simulink model "Flight_Physics_forTrim"  (R2017b)
settings: Solver=ode4  StartTime=0  StopTime=50  FixedStep=Ts  RelTol=1e-3
undefined symbols (not defined in the file or in its folder): Configuration, FOR_LDG_R_B, g, MOM_LDG_R_B, Sim_Control, Ts
libraries: MathLibrary x3, shared6dof x1
settings Model: Creator=zht  LastModifiedBy=zht
settings DataIOCC: SaveFormat=StructureWithTime
settings OptimizationCC: BlockReduction=off  OptimizeBlockIOStorage=off  BufferReuse=off  GlobalBufferReuse=off  ExpressionFolding=off  LocalBlockOutputs=off
settings DebuggingCC: AlgebraicLoopMsg=none  UnconnectedInputMsg=none  UnconnectedOutputMsg=none  UnconnectedLineMsg=none

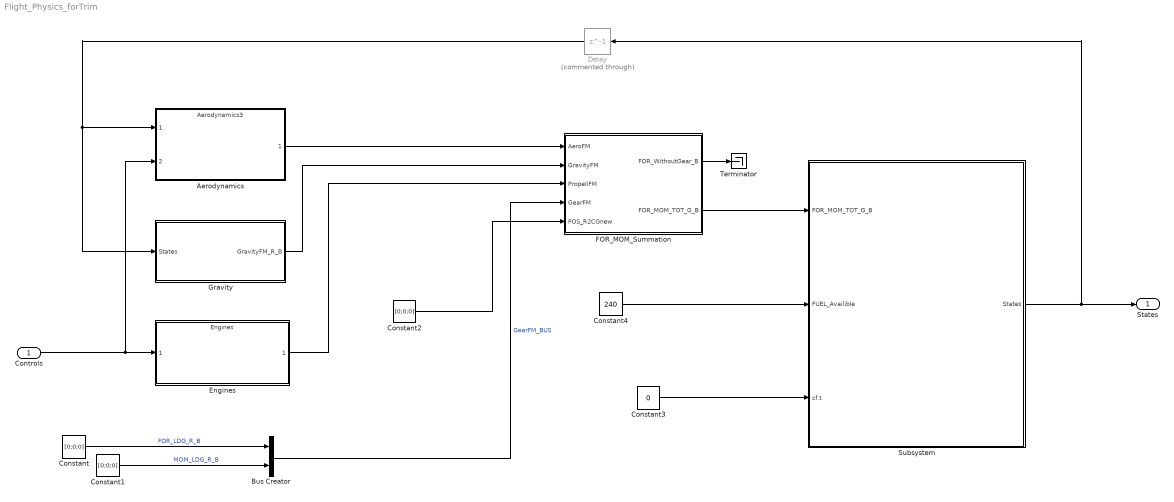
== system Flight_Physics_forTrim ==
  Controls : Inport  OutDataTypeStr=Bus: Controls_CMD_BUS
  Aerodynamics : ModelReference  ModelNameDialog=Aerodynamics3.slx  SimulationMode=Normal  ModelReferenceVersion=1.35
  Bus Creator : BusCreator  Inputs=FOR_LDG_R_B,MOM_LDG_R_B  OutDataTypeStr=Bus: GearFM_BUS  NonVirtualBus=on
  Constant : Constant  Value=[0;0;0]
  Constant1 : Constant  Value=[0;0;0]
  Constant2 : Constant  Value=[0;0;0]
  Constant3 : Constant  Value=0
  Constant4 : Constant  Value=240
  Delay : Delay  Commented=through  DelayLength=1
  Engines : ModelReference  ModelNameDialog=Engines.slx  SimulationMode=Normal  ModelReferenceVersion=1.20
  FOR_MOM_Summation : Subsystem
  Gravity : Subsystem
  Subsystem : Subsystem
  Terminator : Terminator
  States : Outport  OutDataTypeStr=Bus: States_BUS
  wires:
  Controls/1 -> Aerodynamics/2, Engines/1
  Subsystem/1(States) -> States/1, Delay/1
  FOR_MOM_Summation/2(FOR_MOM_TOT_G_B) -> Subsystem/1(FOR_MOM_TOT_G_B)
  Aerodynamics/1 -> FOR_MOM_Summation/1(AeroFM)
  Gravity/1(GravityFM_R_B) -> FOR_MOM_Summation/2(GravityFM)
  Engines/1 -> FOR_MOM_Summation/3(PropellFM)
  Constant4/1 -> Subsystem/2(FUEL_Availible)
  Constant2/1 -> FOR_MOM_Summation/5(POS_R2CGnew)
  Delay/1 -> Gravity/1(States), Aerodynamics/1
  Constant1/1 -> Bus Creator/2  "MOM_LDG_R_B"
  Constant/1 -> Bus Creator/1  "FOR_LDG_R_B"
  Bus Creator/1 -> FOR_MOM_Summation/4(GearFM)  "GearFM_BUS"
  FOR_MOM_Summation/1(FOR_WithoutGear_B) -> Terminator/1
  Constant3/1 -> Subsystem/3(cf.t)

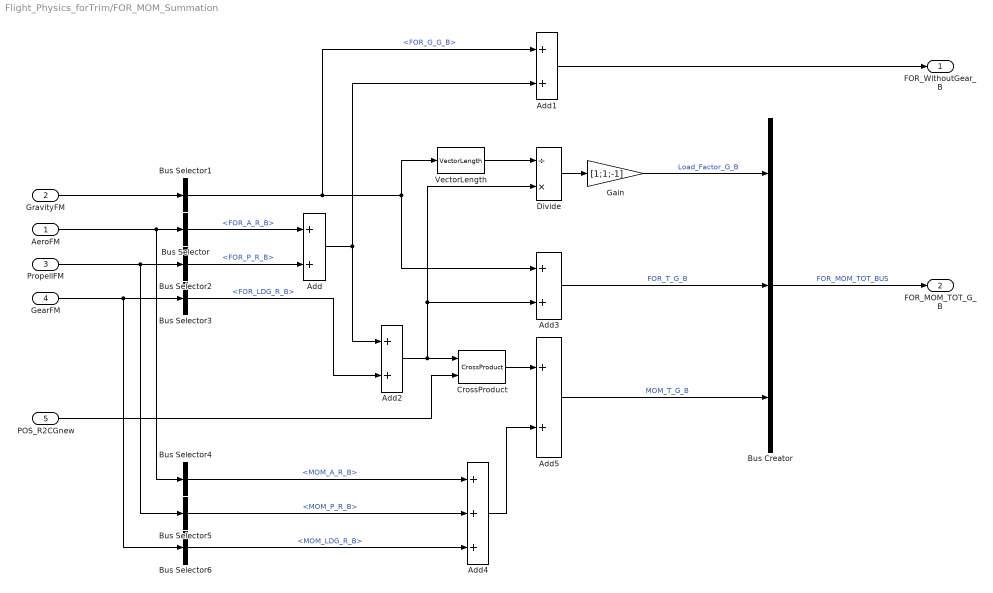
== system Flight_Physics_forTrim/FOR_MOM_Summation ==
  AeroFM : Inport  OutDataTypeStr=Bus: AeroFM_BUS
  GravityFM : Inport  Port=2  OutDataTypeStr=Bus: GravityFM_BUS
  PropellFM : Inport  Port=3  OutDataTypeStr=Bus: PropellFM_BUS
  GearFM : Inport  Port=4  OutDataTypeStr=Bus: GearFM_BUS
  POS_R2CGnew : Inport  Port=5
  Add{,1..3,5} (5 alike) : Sum
  Add4 : Sum  Inputs=+++
  Bus Creator : BusCreator  Inputs=3  OutDataTypeStr=Bus: FOR_MOM_TOT_BUS
  Bus Selector : BusSelector  OutputSignals=FOR_A_R_B
  Bus Selector1 : BusSelector  OutputSignals=FOR_G_G_B
  Bus Selector2 : BusSelector  OutputSignals=FOR_P_R_B
  Bus Selector3 : BusSelector  OutputSignals=FOR_LDG_R_B
  Bus Selector4 : BusSelector  OutputSignals=MOM_A_R_B
  Bus Selector5 : BusSelector  OutputSignals=MOM_P_R_B
  Bus Selector6 : BusSelector  OutputSignals=MOM_LDG_R_B
  CrossProduct : MathLibrary/CrossProduct
  Divide : Product  Inputs=/*
  Gain : Gain  Gain=[1;1;-1]
  VectorLength : MathLibrary/VectorLength
  FOR_WithoutGear_B : Outport
  FOR_MOM_TOT_G_B : Outport  Port=2  OutDataTypeStr=Bus: FOR_MOM_TOT_BUS
  wires:
  PropellFM/1 -> Bus Selector5/1, Bus Selector2/1
  AeroFM/1 -> Bus Selector4/1, Bus Selector/1
  GravityFM/1 -> Bus Selector1/1
  GearFM/1 -> Bus Selector3/1, Bus Selector6/1
  Bus Creator/1 -> FOR_MOM_TOT_G_B/1  "FOR_MOM_TOT_BUS"
  Add1/1 -> FOR_WithoutGear_B/1
  Bus Selector/1 -> Add/1  "<FOR_A_R_B>"
  Bus Selector2/1 -> Add/2  "<FOR_P_R_B>"
  Add/1 -> Add2/1, Add1/2
  Bus Selector1/1 -> Add1/1, VectorLength/1, Add3/1  "<FOR_G_G_B>"
  Bus Selector3/1 -> Add2/2  "<FOR_LDG_R_B>"
  Add2/1 -> CrossProduct/1, Divide/2, Add3/2
  VectorLength/1 -> Divide/1
  Divide/1 -> Gain/1
  Gain/1 -> Bus Creator/1  "Load_Factor_G_B"
  Add3/1 -> Bus Creator/2  "FOR_T_G_B"
  Bus Selector4/1 -> Add4/1  "<MOM_A_R_B>"
  Bus Selector5/1 -> Add4/2  "<MOM_P_R_B>"
  Bus Selector6/1 -> Add4/3  "<MOM_LDG_R_B>"
  CrossProduct/1 -> Add5/1
  Add4/1 -> Add5/2
  Add5/1 -> Bus Creator/3  "MOM_T_G_B"
  POS_R2CGnew/1 -> CrossProduct/2

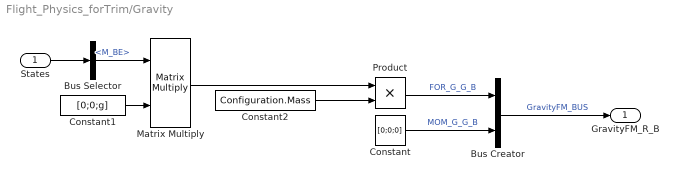
== system Flight_Physics_forTrim/Gravity ==
  States : Inport  OutDataTypeStr=Bus: States_BUS
  Bus Creator : BusCreator  Inputs=2  OutDataTypeStr=Bus: GravityFM_BUS
  Bus Selector : BusSelector  OutputSignals=M_BE
  Constant : Constant  Value=[0;0;0]
  Constant1 : Constant  Value=[0;0;g]  SampleTime=Ts
  Constant2 : Constant  Value=Configuration.Mass  SampleTime=Ts
  Matrix Multiply : Product  Multiplication=Matrix(*)
  Product : Product
  GravityFM_R_B : Outport  OutDataTypeStr=Bus: GravityFM_BUS
  wires:
  States/1 -> Bus Selector/1
  Bus Selector/1 -> Matrix Multiply/1  "<M_BE>"
  Constant1/1 -> Matrix Multiply/2
  Matrix Multiply/1 -> Product/1
  Constant2/1 -> Product/2
  Product/1 -> Bus Creator/1  "FOR_G_G_B"
  Constant/1 -> Bus Creator/2  "MOM_G_G_B"
  Bus Creator/1 -> GravityFM_R_B/1  "GravityFM_BUS"

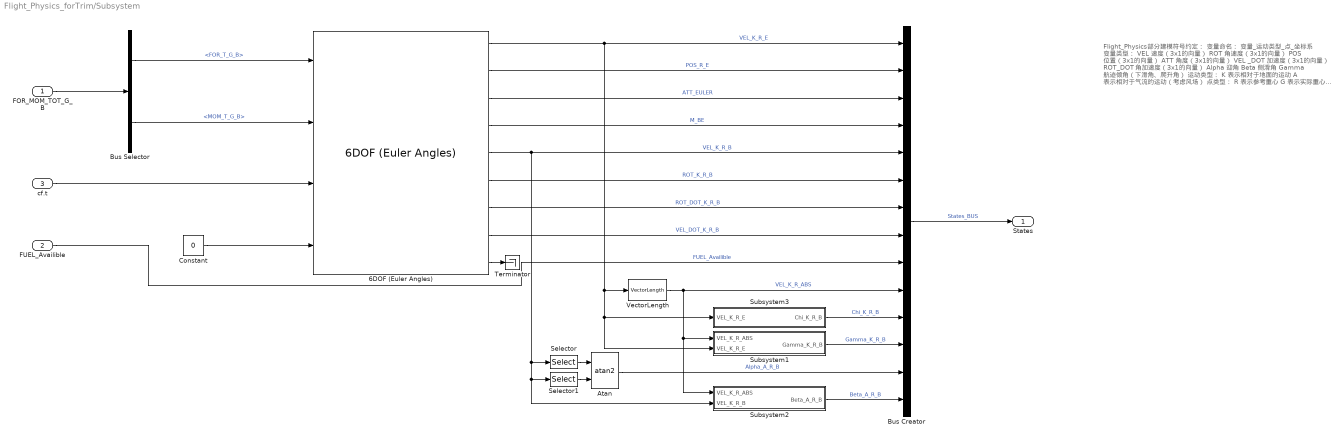
== system Flight_Physics_forTrim/Subsystem ==
  note: Flight_Physics部分建模符号约定：
      | 变量命名：
      | 变量_运动类型_点_坐标系
      |
      | 变量类型：
      | VEL 速度（3x1的向量）
      | ROT 角速度（3x1的向量）
      | POS 位置（3x1的向量）
      | ATT 角度（3x1的向量）
      | VEL _DOT 加速度（3x1的向量）
      | ROT_DOT 角加速度（3x1的向量）
      | Alpha 迎角
      | Beta 侧滑角
      | Gamma 航迹倾角（下滑角、爬升角）
      | 运动类型：
      | K 表示相对于地面的运动
      | A 表示相对于气流的运动（考虑风场）
      | 点类型：
      | R 表示参考重心
      | G 表示实际重心
      | 坐标系类型：
      | B 机体系
      | E 地面系 ABS 与坐标系无关，表示该变量的绝对值
  FOR_MOM_TOT_G_B : Inport  OutDataTypeStr=Bus: FOR_MOM_TOT_BUS
  FUEL_Availible : Inport  Port=2
  cf.t : Inport  Port=3
  6DOF (Euler Angles) : shared6dof/6DOF (Euler Angles)  units=Metric (MKS)  mtype=Simple Variable  rep=Euler Angles  xme_0=Sim_Control.init(1,:)  Vm_0=Sim_Control.init(2,:)  eul_0=Sim_Control.init(3,:)  pm_0=Sim_Control.init(4,:)  mass_0=Configuration.Mass  mass_e=Configuration.Mass_Constr  mass_f=Configuration.Mass  inertia=eye(3)  inertia_e=Configuration.Inertia_G_B  inertia_f=Configuration.Inertia_G_B  k_quat=1.0  vre_flag=on  abi_flag=off
      settings: SourceProductBaseCode=AE
  Atan : Trigonometry  Operator=atan2
  Bus Creator : BusCreator  Inputs=14  OutDataTypeStr=Bus: States_BUS
  Bus Selector : BusSelector  OutputSignals=FOR_T_G_B,MOM_T_G_B
  Constant : Constant  Value=0
  Selector : Selector  InputPortWidth=3  IndexOptions=Index vector (dialog)  Indices=[3]  OutputSizes=1
  Selector1 : Selector  InputPortWidth=3  IndexOptions=Index vector (dialog)  Indices=[1]  OutputSizes=1
  Subsystem1 : Subsystem
  Subsystem2 : Subsystem
  Subsystem3 : Subsystem
  Terminator : Terminator
  VectorLength : MathLibrary/VectorLength
  States : Outport  OutDataTypeStr=Bus: States_BUS
  wires:
  Bus Creator/1 -> States/1  "States_BUS"
  Bus Selector/2 -> 6DOF (Euler Angles)/2  "<MOM_T_G_B>"
  Bus Selector/1 -> 6DOF (Euler Angles)/1  "<FOR_T_G_B>"
  FOR_MOM_TOT_G_B/1 -> Bus Selector/1
  6DOF (Euler Angles)/1 -> VectorLength/1, Subsystem3/1(VEL_K_R_E), Subsystem1/2(VEL_K_R_E), Bus Creator/1  "VEL_K_R_E"
  6DOF (Euler Angles)/2 -> Bus Creator/2  "POS_R_E"
  6DOF (Euler Angles)/3 -> Bus Creator/3  "ATT_EULER"
  6DOF (Euler Angles)/4 -> Bus Creator/4  "M_BE"
  6DOF (Euler Angles)/5 -> Subsystem2/2(VEL_K_R_B), Selector1/1, Selector/1, Bus Creator/5  "VEL_K_R_B"
  6DOF (Euler Angles)/6 -> Bus Creator/6  "ROT_K_R_B"
  6DOF (Euler Angles)/7 -> Bus Creator/7  "ROT_DOT_K_R_B"
  6DOF (Euler Angles)/8 -> Bus Creator/8  "VEL_DOT_K_R_B"
  FUEL_Availible/1 -> Bus Creator/9  "FUEL_Availible"
  Selector/1 -> Atan/1
  Selector1/1 -> Atan/2
  Atan/1 -> Bus Creator/13  "Alpha_A_R_B"
  VectorLength/1 -> Subsystem1/1(VEL_K_R_ABS), Subsystem2/1(VEL_K_R_ABS), Bus Creator/10  "VEL_K_R_ABS"
  Subsystem1/1(Gamma_K_R_B) -> Bus Creator/12  "Gamma_K_R_B"
  Subsystem2/1(Beta_A_R_B) -> Bus Creator/14  "Beta_A_R_B"
  Subsystem3/1(Chi_K_R_B) -> Bus Creator/11  "Chi_K_R_B"
  Constant/1 -> 6DOF (Euler Angles)/4
  cf.t/1 -> 6DOF (Euler Angles)/3
  6DOF (Euler Angles)/9 -> Terminator/1

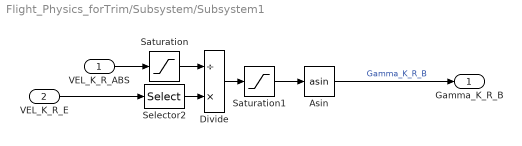
== system Flight_Physics_forTrim/Subsystem/Subsystem1 ==
  VEL_K_R_ABS : Inport
  VEL_K_R_E : Inport  Port=2
  Asin : Trigonometry  Operator=asin
  Divide : Product  Inputs=/*
  Saturation : Saturate  UpperLimit=inf  LowerLimit=0.01
  Saturation1 : Saturate  UpperLimit=1  LowerLimit=-1
  Selector2 : Selector  InputPortWidth=3  IndexOptions=Index vector (dialog)  Indices=[3]  OutputSizes=1
  Gamma_K_R_B : Outport
  wires:
  Divide/1 -> Saturation1/1
  Asin/1 -> Gamma_K_R_B/1  "Gamma_K_R_B"
  VEL_K_R_E/1 -> Selector2/1
  VEL_K_R_ABS/1 -> Saturation/1
  Selector2/1 -> Divide/2
  Saturation1/1 -> Asin/1
  Saturation/1 -> Divide/1

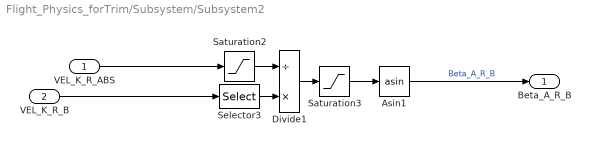
== system Flight_Physics_forTrim/Subsystem/Subsystem2 ==
  VEL_K_R_ABS : Inport
  VEL_K_R_B : Inport  Port=2
  Asin1 : Trigonometry  Operator=asin
  Divide1 : Product  Inputs=/*
  Saturation2 : Saturate  UpperLimit=inf  LowerLimit=0.01
  Saturation3 : Saturate  UpperLimit=1  LowerLimit=-1
  Selector3 : Selector  InputPortWidth=3  IndexOptions=Index vector (dialog)  Indices=[2]  OutputSizes=1
  Beta_A_R_B : Outport
  wires:
  Saturation2/1 -> Divide1/1
  Asin1/1 -> Beta_A_R_B/1  "Beta_A_R_B"
  Saturation3/1 -> Asin1/1
  Selector3/1 -> Divide1/2
  Divide1/1 -> Saturation3/1
  VEL_K_R_B/1 -> Selector3/1
  VEL_K_R_ABS/1 -> Saturation2/1

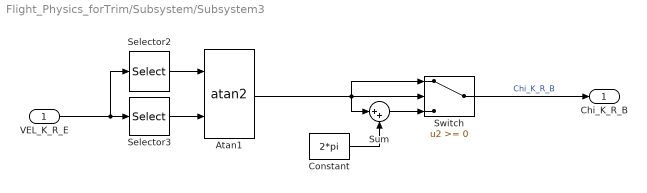
== system Flight_Physics_forTrim/Subsystem/Subsystem3 ==
  VEL_K_R_E : Inport
  Atan1 : Trigonometry  Operator=atan2
  Constant : Constant  Value=2*pi
  Selector2 : Selector  InputPortWidth=3  IndexOptions=Index vector (dialog)  Indices=[2]  OutputSizes=1
  Selector3 : Selector  InputPortWidth=3  IndexOptions=Index vector (dialog)  Indices=[1]  OutputSizes=1
  Sum : Sum  Inputs=|++
  Switch : Switch
  Chi_K_R_B : Outport
  wires:
  Selector2/1 -> Atan1/1
  Selector3/1 -> Atan1/2
  VEL_K_R_E/1 -> Selector2/1, Selector3/1
  Switch/1 -> Chi_K_R_B/1  "Chi_K_R_B"
  Atan1/1 -> Sum/1, Switch/1, Switch/2
  Constant/1 -> Sum/2
  Sum/1 -> Switch/3
